simulink model "gm_RLUb_HIL"  (R2018b)
settings: Solver=VariableStepAuto  StartTime=0.0  StopTime=15e-3  RelTol=1e-6  EnableMultiTasking=on
undefined symbols (not defined in the file or in its folder): dt, I_FS, L, R, U_FS
libraries: simulink x53, hdlmdlgenlib x11, hdlsllib x9
settings Model: Creator=suti  LastModifiedBy=natlo
settings DataIOCC: LimitDataPoints=on  SaveFormat=Array  SaveOutput=off  SaveTime=off
settings OptimizationCC: BlockReduction=off  ConditionallyExecuteInputs=off  DefaultParameterBehavior=Inlined  ExpressionDepthLimit=2147483647  LifeSpan=1
settings DebuggingCC: AlgebraicLoopMsg=error  UnderspecifiedInitializationDetection=Classic  MergeDetectMultiDrivingBlocksExec=none  SolverPrmCheckMsg=warning  InheritedTsInSrcMsg=none  FcnCallInpInsideContextMsg=warning  StateNameClashWarn=warning  SFUnexpectedBacktrackingDiag=warning  SFNoUnconditionalDefaultTransitionDiag=warning  SFExecutionAtInitializationDiag=none
settings HardwareCC: ProdBitPerPointer=32  ProdBitPerSizeT=32  ProdBitPerPtrDiffT=32  ProdLargestAtomicFloat=None  ProdIntDivRoundTo=Undefined  ProdEndianess=Unspecified  ProdWordSize=32  ProdHWDeviceType=ASIC/FPGA->ASIC/FPGA  TargetBitPerPointer=64  TargetBitPerSizeT=64  TargetBitPerPtrDiffT=64  TargetLongLongMode=on  TargetIntDivRoundTo=Zero  TargetEndianess=LittleEndian  TargetWordSize=64  TargetHWDeviceType=Custom Processor->MATLAB Host Computer  ProdEqTarget=off
settings ModelReferenceCC: PropagateSignalLabelsOutOfModel=off
settings SFSimCC: SimUseLocalCustomCode=off
settings RTWCC: RTWUseLocalCustomCode=off
settings CodeAppCC: StateflowObjectComments=on
settings GRTTargetCC: TargetLangStandard=C89/C90 (ANSI)  GeneratePreprocessorConditionals=Disable all  CombineOutputUpdateFcns=off  GRTInterface=on
settings ConfigComp: CovMetricSettings=dw  CovHtmlReporting=on  CovSaveCumulativeToWorkspaceVar=on  CovSaveSingleToWorkspaceVar=on  CovExternalEMLEnable=off  CovSFcnEnable=off

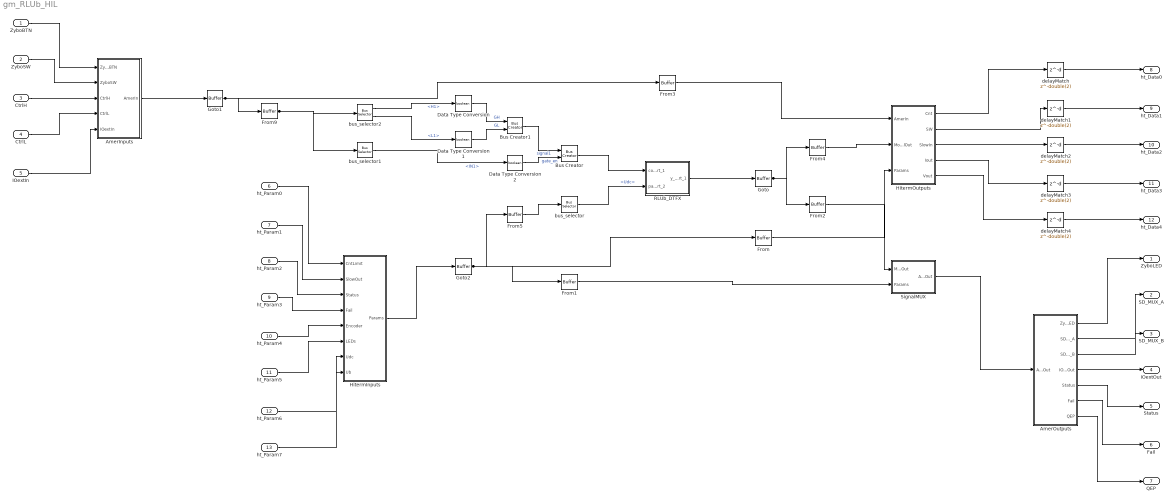
== system gm_RLUb_HIL ==
  ZyboBTN : Inport  OutDataTypeStr=fixdt(0, 3, 0)  PortDimensions=1  SampleTime=5e-08
  ZyboSW : Inport  Port=2  OutDataTypeStr=fixdt(0, 4, 0)  PortDimensions=1  SampleTime=5e-08
  CtrlH : Inport  Port=3  OutDataTypeStr=fixdt(0, 4, 0)  PortDimensions=1  SampleTime=5e-08
  CtrlL : Inport  Port=4  OutDataTypeStr=fixdt(0, 4, 0)  PortDimensions=1  SampleTime=5e-08
  IOextIn : Inport  Port=5  OutDataTypeStr=uint8  PortDimensions=1  SampleTime=5e-08
  ht_Param0 : Inport  Port=6  OutDataTypeStr=uint32  PortDimensions=1  SampleTime=5e-08
  ht_Param1 : Inport  Port=7  OutDataTypeStr=uint32  PortDimensions=1  SampleTime=5e-08
  ht_Param2 : Inport  Port=8  OutDataTypeStr=uint32  PortDimensions=1  SampleTime=5e-08
  ht_Param3 : Inport  Port=9  OutDataTypeStr=uint32  PortDimensions=1  SampleTime=5e-08
  ht_Param4 : Inport  Port=10  OutDataTypeStr=uint32  PortDimensions=1  SampleTime=5e-08
  ht_Param5 : Inport  Port=11  OutDataTypeStr=uint32  PortDimensions=1  SampleTime=5e-08
  ht_Param6 : Inport  Port=12  OutDataTypeStr=uint32  PortDimensions=1  SampleTime=5e-08
  ht_Param7 : Inport  Port=13  OutDataTypeStr=uint32  PortDimensions=1  SampleTime=5e-08
  AmerInputs : Subsystem
  AmerOutputs : Subsystem
  Bus Creator : BusCreator  Inputs=2
  Bus Creator1 : BusCreator  Inputs=2
  Data Type Conversion : DataTypeConversion  OutDataTypeStr=boolean  SampleTime=5e-08
  Data Type Conversion1 : DataTypeConversion  OutDataTypeStr=boolean  SampleTime=5e-08
  Data Type Conversion2 : DataTypeConversion  OutDataTypeStr=boolean  SampleTime=5e-08
  From{,1..5,9} (7 alike) : hdlmdlgenlib/Buffer
      settings: SourceProductName=HDL Coder  SourceProductBaseCode=HD
  Goto : hdlmdlgenlib/Buffer
      settings: SourceProductName=HDL Coder  SourceProductBaseCode=HD
  Goto1 : hdlmdlgenlib/Buffer
      settings: SourceProductName=HDL Coder  SourceProductBaseCode=HD
  Goto2 : hdlmdlgenlib/Buffer
      settings: SourceProductName=HDL Coder  SourceProductBaseCode=HD
  HitermInputs : Subsystem
  HitermOutputs : Subsystem
  RLUb_DTFX : Subsystem
  SignalMUX : Subsystem
  bus_selector : BusSelector  OutputSignals=Udc,Ub  OutputAsBus=on
  bus_selector1 : BusSelector  OutputSignals=SlowIn.IN1  OutputAsBus=on
  bus_selector2 : BusSelector  OutputSignals=Ctrl.GH.H1,Ctrl.GL.L1
  delayMatch{,1..4} (5 alike) : Delay  DelayLength=double(2)  InitialCondition=0  InputProcessing=Inherited  SampleTime=5e-08
  ZyboLED : Outport  SampleTime=dt
  SD_MUX_A : Outport  Port=2  SampleTime=dt
  SD_MUX_B : Outport  Port=3  SampleTime=dt
  IOextOut : Outport  Port=4
  Status : Outport  Port=5
  Fail : Outport  Port=6
  QEP : Outport  Port=7
  ht_Data0 : Outport  Port=8
  ht_Data1 : Outport  Port=9
  ht_Data2 : Outport  Port=10
  ht_Data3 : Outport  Port=11
  ht_Data4 : Outport  Port=12
  wires:
  ZyboBTN/1 -> AmerInputs/1(ZyboBTN)
  ZyboSW/1 -> AmerInputs/2(ZyboSW)
  CtrlH/1 -> AmerInputs/3(CtrlH)
  CtrlL/1 -> AmerInputs/4(CtrlL)
  IOextIn/1 -> AmerInputs/5(IOextIn)
  ht_Param0/1 -> HitermInputs/1(CntLimit)
  ht_Param1/1 -> HitermInputs/2(SlowOut)
  ht_Param2/1 -> HitermInputs/3(Status)
  ht_Param3/1 -> HitermInputs/4(Fail)
  ht_Param4/1 -> HitermInputs/5(Encoder)
  ht_Param5/1 -> HitermInputs/6(LEDs)
  ht_Param6/1 -> HitermInputs/7(Udc)
  ht_Param7/1 -> HitermInputs/8(Ub)
  AmerInputs/1(AmerIn) -> Goto1/1
  AmerOutputs/1(ZyboLED) -> ZyboLED/1
  AmerOutputs/2(SD_MUX_A) -> SD_MUX_A/1
  AmerOutputs/3(SD_MUX_B) -> SD_MUX_B/1
  AmerOutputs/4(IOextOut) -> IOextOut/1
  AmerOutputs/5(Status) -> Status/1
  AmerOutputs/6(Fail) -> Fail/1
  AmerOutputs/7(QEP) -> QEP/1
  Bus Creator/1 -> RLUb_DTFX/1(control_Inport_1)
  Bus Creator1/1 -> Bus Creator/1  "signal1"
  bus_selector/1 -> RLUb_DTFX/2(par_Inport_2)  "<Udc>"
  bus_selector1/1 -> Data Type Conversion2/1  "<IN1>"
  bus_selector2/1 -> Data Type Conversion/1  "<H1>"
  bus_selector2/2 -> Data Type Conversion1/1  "<L1>"
  Data Type Conversion/1 -> Bus Creator1/1  "GH"
  Data Type Conversion1/1 -> Bus Creator1/2  "GL"
  Data Type Conversion2/1 -> Bus Creator/2  "gate_en"
  From/1 -> HitermOutputs/3(Params)
  From1/1 -> SignalMUX/2(Params)
  From2/1 -> SignalMUX/1(ModelOut)
  From3/1 -> HitermOutputs/1(AmerIn)
  From4/1 -> HitermOutputs/2(ModelOut)
  From5/1 -> bus_selector/1
  From9/1 -> bus_selector2/1, bus_selector1/1
  HitermInputs/1(Params) -> Goto2/1
  delayMatch/1 -> ht_Data0/1
  delayMatch1/1 -> ht_Data1/1
  delayMatch2/1 -> ht_Data2/1
  delayMatch3/1 -> ht_Data3/1
  delayMatch4/1 -> ht_Data4/1
  RLUb_DTFX/1(y_Outport_1) -> Goto/1
  SignalMUX/1(AmerOut) -> AmerOutputs/1(AmerOut)
  Goto2/1 -> From5/1, From1/1, From/1
  Goto/1 -> From4/1, From2/1
  Goto1/1 -> From9/1, From3/1
  HitermOutputs/1(Cnt) -> delayMatch/1
  HitermOutputs/2(SW) -> delayMatch1/1
  HitermOutputs/3(SlowIn) -> delayMatch2/1
  HitermOutputs/4(Iout) -> delayMatch3/1
  HitermOutputs/5(Vout) -> delayMatch4/1

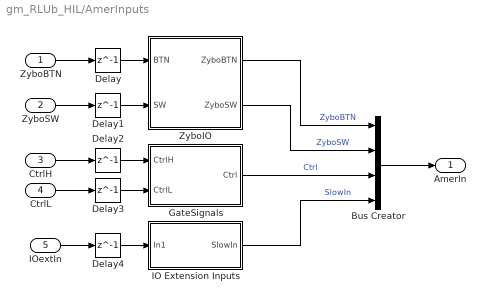
== system gm_RLUb_HIL/AmerInputs ==
  ZyboBTN : Inport  OutDataTypeStr=fixdt(0, 3, 0)  PortDimensions=1  SampleTime=5e-08
  ZyboSW : Inport  Port=2  OutDataTypeStr=fixdt(0, 4, 0)  PortDimensions=1  SampleTime=5e-08
  CtrlH : Inport  Port=3  OutDataTypeStr=fixdt(0, 4, 0)  PortDimensions=1  SampleTime=5e-08
  CtrlL : Inport  Port=4  OutDataTypeStr=fixdt(0, 4, 0)  PortDimensions=1  SampleTime=5e-08
  IOextIn : Inport  Port=5  OutDataTypeStr=uint8  PortDimensions=1  SampleTime=5e-08
  Bus Creator : BusCreator  Inputs=4
  Delay{,1..4} (5 alike) : Delay  DelayLength=1  InitialCondition=0
  GateSignals : Subsystem
  IO Extension Inputs : Subsystem
  ZyboIO : Subsystem
  AmerIn : Outport
  wires:
  Bus Creator/1 -> AmerIn/1
  Delay/1 -> ZyboIO/1(BTN)
  Delay1/1 -> ZyboIO/2(SW)
  Delay2/1 -> GateSignals/1(CtrlH)
  Delay3/1 -> GateSignals/2(CtrlL)
  Delay4/1 -> IO Extension Inputs/1(In1)
  GateSignals/1(Ctrl) -> Bus Creator/3  "Ctrl"
  IO Extension Inputs/1(SlowIn) -> Bus Creator/4  "SlowIn"
  ZyboIO/1(ZyboBTN) -> Bus Creator/1  "ZyboBTN"
  ZyboIO/2(ZyboSW) -> Bus Creator/2  "ZyboSW"
  ZyboBTN/1 -> Delay/1
  ZyboSW/1 -> Delay1/1
  CtrlH/1 -> Delay2/1
  CtrlL/1 -> Delay3/1
  IOextIn/1 -> Delay4/1

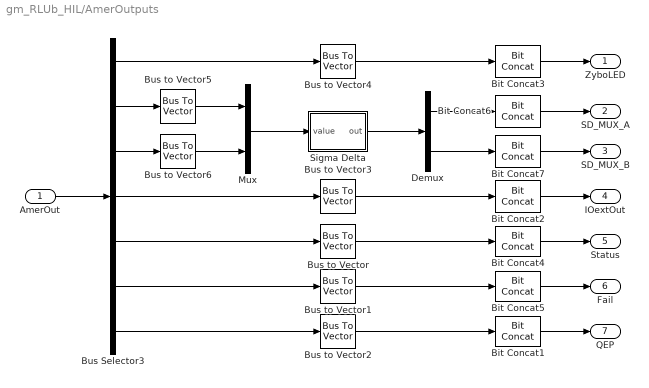
== system gm_RLUb_HIL/AmerOutputs ==
  AmerOut : Inport  SampleTime=5e-08
  Bit Concat{1..7} (7 alike) : hdlsllib/Logic and Bit Operations/Bit Concat  numInputs=1
      settings: SourceProductName=HDL Coder  SourceProductBaseCode=HD
  Bus Selector3 : BusSelector  OutputSignals=ZyboLED,ANA,ANB,SlowOut,Status,Fail,Encoder
  Bus to Vector{,1..6} (7 alike) : BusToVector
  Demux : Demux  Outputs=[8,8]
  Mux : Mux  Inputs=2
  Sigma Delta : Subsystem  mask{N=double(16), dt=double(-1)}
      mask prompts: N "Required resolution (bits)"; dt "Sample time"
  ZyboLED : Outport
  SD_MUX_A : Outport  Port=2  SampleTime=dt
  SD_MUX_B : Outport  Port=3  SampleTime=dt
  IOextOut : Outport  Port=4
  Status : Outport  Port=5
  Fail : Outport  Port=6
  QEP : Outport  Port=7
  wires:
  Bit Concat1/1 -> QEP/1
  Bit Concat2/1 -> IOextOut/1
  Bit Concat3/1 -> ZyboLED/1
  Bit Concat4/1 -> Status/1
  Bit Concat5/1 -> Fail/1
  Bit Concat6/1 -> SD_MUX_A/1
  Bit Concat7/1 -> SD_MUX_B/1
  Bus Selector3/1 -> Bus to Vector4/1
  Bus Selector3/2 -> Bus to Vector5/1
  Bus Selector3/3 -> Bus to Vector6/1
  Bus Selector3/4 -> Bus to Vector3/1
  Bus Selector3/5 -> Bus to Vector/1
  Bus Selector3/6 -> Bus to Vector1/1
  Bus Selector3/7 -> Bus to Vector2/1
  Bus to Vector/1 -> Bit Concat4/1
  Bus to Vector1/1 -> Bit Concat5/1
  Bus to Vector2/1 -> Bit Concat1/1
  Bus to Vector3/1 -> Bit Concat2/1
  Bus to Vector4/1 -> Bit Concat3/1
  Bus to Vector5/1 -> Mux/1
  Bus to Vector6/1 -> Mux/2
  Demux/1 -> Bit Concat6/1
  Demux/2 -> Bit Concat7/1
  Mux/1 -> Sigma Delta/1(value)
  Sigma Delta/1(out) -> Demux/1
  AmerOut/1 -> Bus Selector3/1

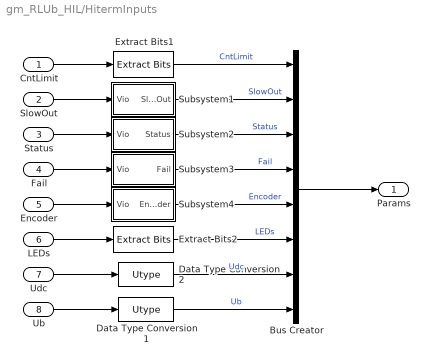
== system gm_RLUb_HIL/HitermInputs ==
  CntLimit : Inport  OutDataTypeStr=uint32  PortDimensions=1  SampleTime=5e-08
  SlowOut : Inport  Port=2  OutDataTypeStr=uint32  PortDimensions=1  SampleTime=5e-08
  Status : Inport  Port=3  OutDataTypeStr=uint32  PortDimensions=1  SampleTime=5e-08
  Fail : Inport  Port=4  OutDataTypeStr=uint32  PortDimensions=1  SampleTime=5e-08
  Encoder : Inport  Port=5  OutDataTypeStr=uint32  PortDimensions=1  SampleTime=5e-08
  LEDs : Inport  Port=6  OutDataTypeStr=uint32  PortDimensions=1  SampleTime=5e-08
  Udc : Inport  Port=7  OutDataTypeStr=uint32  PortDimensions=1  SampleTime=5e-08
  Ub : Inport  Port=8  OutDataTypeStr=uint32  PortDimensions=1  SampleTime=5e-08
  Bus Creator : BusCreator  Inputs=8
  Data Type Conversion1 : DataTypeConversion  OutDataTypeStr=Utype  ConvertRealWorld=Stored Integer (SI)
  Data Type Conversion2 : DataTypeConversion  OutMin=[0]  OutDataTypeStr=Utype  ConvertRealWorld=Stored Integer (SI)
  Extract Bits1 : simulink/Logic and Bit Operations/Extract Bits  bitsToExtract=Range of bits  numBits=8  bitIdxRange=[0 15]  outScalingMode=Treat bit field as an integer
      settings: SourceProductName=Simulink
  Extract Bits2 : simulink/Logic and Bit Operations/Extract Bits  bitsToExtract=Range of bits  numBits=8  bitIdxRange=[0 3]  outScalingMode=Treat bit field as an integer
      settings: SourceProductName=Simulink
  Subsystem1 : Subsystem
  Subsystem2 : Subsystem
  Subsystem3 : Subsystem
  Subsystem4 : Subsystem
  Params : Outport
  wires:
  Bus Creator/1 -> Params/1
  Data Type Conversion1/1 -> Bus Creator/8  "Ub"
  Data Type Conversion2/1 -> Bus Creator/7  "Udc"
  Extract Bits1/1 -> Bus Creator/1  "CntLimit"
  Extract Bits2/1 -> Bus Creator/6  "LEDs"
  Subsystem1/1(SlowOut) -> Bus Creator/2  "SlowOut"
  Subsystem2/1(Status) -> Bus Creator/3  "Status"
  Subsystem3/1(Fail) -> Bus Creator/4  "Fail"
  Subsystem4/1(Encoder) -> Bus Creator/5  "Encoder"
  CntLimit/1 -> Extract Bits1/1
  SlowOut/1 -> Subsystem1/1(Vio)
  Status/1 -> Subsystem2/1(Vio)
  Fail/1 -> Subsystem3/1(Vio)
  Encoder/1 -> Subsystem4/1(Vio)
  LEDs/1 -> Extract Bits2/1
  Udc/1 -> Data Type Conversion2/1
  Ub/1 -> Data Type Conversion1/1

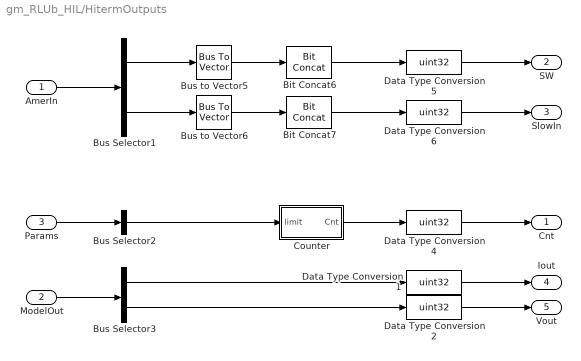
== system gm_RLUb_HIL/HitermOutputs ==
  AmerIn : Inport  SampleTime=5e-08
  ModelOut : Inport  Port=2  SampleTime=5e-08
  Params : Inport  Port=3  SampleTime=5e-08
  Bit Concat6 : hdlsllib/Logic and Bit Operations/Bit Concat  numInputs=1
      settings: SourceProductName=HDL Coder  SourceProductBaseCode=HD
  Bit Concat7 : hdlsllib/Logic and Bit Operations/Bit Concat  numInputs=1
      settings: SourceProductName=HDL Coder  SourceProductBaseCode=HD
  Bus Selector1 : BusSelector  OutputSignals=ZyboSW,SlowIn
  Bus Selector2 : BusSelector  OutputSignals=CntLimit
  Bus Selector3 : BusSelector  OutputSignals=Iout,Vout
  Bus to Vector5 : BusToVector
  Bus to Vector6 : BusToVector
  Counter : Subsystem
  Data Type Conversion1 : DataTypeConversion  OutDataTypeStr=uint32  ConvertRealWorld=Stored Integer (SI)
  Data Type Conversion2 : DataTypeConversion  OutDataTypeStr=uint32  ConvertRealWorld=Stored Integer (SI)
  Data Type Conversion4 : DataTypeConversion  OutDataTypeStr=uint32
  Data Type Conversion5 : DataTypeConversion  OutDataTypeStr=uint32
  Data Type Conversion6 : DataTypeConversion  OutDataTypeStr=uint32
  Cnt : Outport
  SW : Outport  Port=2
  SlowIn : Outport  Port=3
  Iout : Outport  Port=4
  Vout : Outport  Port=5
  wires:
  Bit Concat6/1 -> Data Type Conversion5/1
  Bit Concat7/1 -> Data Type Conversion6/1
  Bus Selector1/1 -> Bus to Vector5/1
  Bus Selector1/2 -> Bus to Vector6/1
  Bus Selector2/1 -> Counter/1(limit)
  Bus Selector3/1 -> Data Type Conversion1/1
  Bus Selector3/2 -> Data Type Conversion2/1
  Bus to Vector5/1 -> Bit Concat6/1
  Bus to Vector6/1 -> Bit Concat7/1
  Counter/1(Cnt) -> Data Type Conversion4/1
  Data Type Conversion1/1 -> Iout/1
  Data Type Conversion2/1 -> Vout/1
  Data Type Conversion4/1 -> Cnt/1
  Data Type Conversion5/1 -> SW/1
  Data Type Conversion6/1 -> SlowIn/1
  AmerIn/1 -> Bus Selector1/1
  ModelOut/1 -> Bus Selector3/1
  Params/1 -> Bus Selector2/1

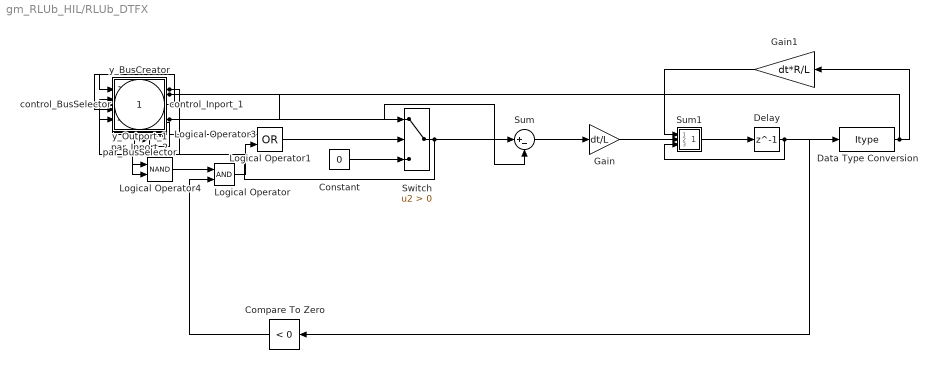
== system gm_RLUb_HIL/RLUb_DTFX ==
  control_Inport_1 : Inport  SampleTime=5e-08
  par_Inport_2 : Inport  Port=2  SampleTime=5e-08
  Compare To Zero : simulink/Logic and Bit Operations/Compare To Zero  relop=<  OutDataTypeStr=boolean
  Constant : Constant  Value=0  OutDataTypeStr=Inherit: Inherit via back propagation  SampleTime=-1
  Data Type Conversion : DataTypeConversion  OutDataTypeStr=Itype
  Delay : Delay  DelayLength=1
  Gain : Gain  Gain=dt/L  OutMax=[2*U_FS*dt/L]  OutDataTypeStr=fixdt(1,vbits)
  Gain1 : Gain  Gain=dt*R/L  OutMax=[I_FS*dt*R/L]  OutDataTypeStr=fixdt(1,vbits)
  Logical Operator : Logic  IconShape=distinctive  AllPortsSameDT=off  OutDataTypeStr=boolean
  Logical Operator1 : Logic  Operator=OR  IconShape=distinctive  AllPortsSameDT=off  OutDataTypeStr=boolean
  Logical Operator3 : Logic  IconShape=distinctive  AllPortsSameDT=off  OutDataTypeStr=boolean
  Logical Operator4 : Logic  Operator=NAND  IconShape=distinctive  AllPortsSameDT=off  OutDataTypeStr=boolean
  Sum : Sum  Inputs=|+-  OutDataTypeStr=Inherit: Same as accumulator
  Sum1 : Subsystem
  Switch : Switch  Criteria=u2 > Threshold
  control_BusSelector : Subsystem
  par_BusSelector : Subsystem
  y_BusCreator : Subsystem
  y_Outport_1 : Outport
  wires:
  Constant/1 -> Switch/3
  Data Type Conversion/1 -> y_BusCreator/1(y_BusCreator_In1), Gain1/1
  Logical Operator3/1 -> Logical Operator1/1
  Logical Operator4/1 -> Logical Operator/1
  Switch/1 -> y_BusCreator/2(y_BusCreator_In2), Sum/1
  control_BusSelector/1(control_BusSelector_Out1) -> Logical Operator4/2, Logical Operator3/2
  control_BusSelector/2(control_BusSelector_Out2) -> Logical Operator3/1
  control_BusSelector/3(control_BusSelector_Out3) -> Logical Operator4/1
  par_BusSelector/1(par_BusSelector_Out1) -> y_BusCreator/3(y_BusCreator_In3), Switch/1
  par_BusSelector/2(par_BusSelector_Out2) -> y_BusCreator/4(y_BusCreator_In4), Sum/2
  y_BusCreator/1(y_BusCreator_Out1) -> y_Outport_1/1
  control_Inport_1/1 -> control_BusSelector/1(control_BusSelector_In1)
  par_Inport_2/1 -> par_BusSelector/1(par_BusSelector_In1)
  Compare To Zero/1 -> Logical Operator/2
  Logical Operator/1 -> Logical Operator1/2
  Logical Operator1/1 -> Switch/2
  Sum/1 -> Gain/1
  Gain/1 -> Sum1/2(In2)
  Gain1/1 -> Sum1/1(In1)
  Sum1/1(Out1) -> Delay/1
  Delay/1 -> Sum1/3(In3), Data Type Conversion/1, Compare To Zero/1

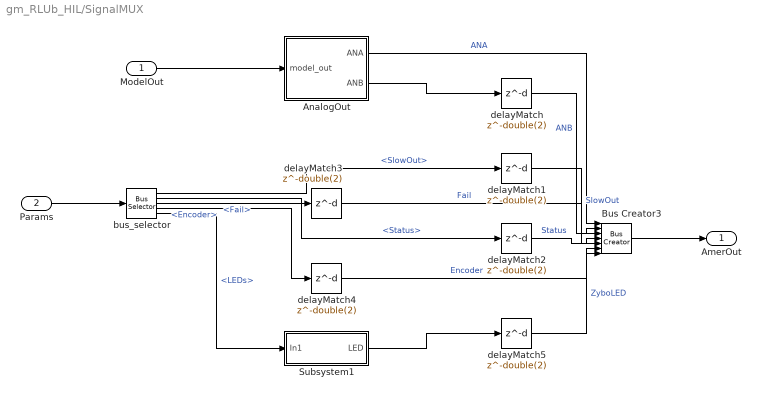
== system gm_RLUb_HIL/SignalMUX ==
  ModelOut : Inport  SampleTime=5e-08
  Params : Inport  Port=2  SampleTime=5e-08
  AnalogOut : Subsystem
  Bus Creator3 : BusCreator  Inputs=7
  Subsystem1 : Subsystem
  bus_selector : BusSelector  OutputSignals=SlowOut,Status,Fail,Encoder,LEDs
  delayMatch{,1..5} (6 alike) : Delay  DelayLength=double(2)  InitialCondition=0  InputProcessing=Inherited  SampleTime=5e-08
  AmerOut : Outport
  wires:
  AnalogOut/1(ANA) -> Bus Creator3/1  "ANA"
  delayMatch/1 -> Bus Creator3/2  "ANB"
  Bus Creator3/1 -> AmerOut/1
  delayMatch1/1 -> Bus Creator3/3  "SlowOut"
  delayMatch2/1 -> Bus Creator3/4  "Status"
  delayMatch3/1 -> Bus Creator3/5  "Fail"
  delayMatch4/1 -> Bus Creator3/6  "Encoder"
  bus_selector/5 -> Subsystem1/1(In1)  "<LEDs>"
  delayMatch5/1 -> Bus Creator3/7  "ZyboLED"
  ModelOut/1 -> AnalogOut/1(model_out)
  Params/1 -> bus_selector/1
  AnalogOut/2(ANB) -> delayMatch/1
  bus_selector/1 -> delayMatch1/1  "<SlowOut>"
  bus_selector/2 -> delayMatch2/1  "<Status>"
  bus_selector/3 -> delayMatch3/1  "<Fail>"
  bus_selector/4 -> delayMatch4/1  "<Encoder>"
  Subsystem1/1(LED) -> delayMatch5/1

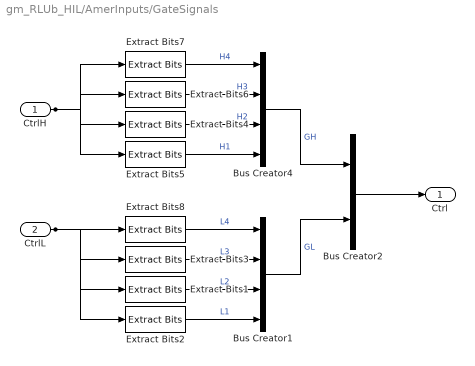
== system gm_RLUb_HIL/AmerInputs/GateSignals ==
  CtrlH : Inport  OutDataTypeStr=fixdt(0, 4, 0)  PortDimensions=1  SampleTime=5e-08
  CtrlL : Inport  Port=2  OutDataTypeStr=fixdt(0, 4, 0)  PortDimensions=1  SampleTime=5e-08
  Bus Creator1 : BusCreator  Inputs=4
  Bus Creator2 : BusCreator  Inputs=2
  Bus Creator4 : BusCreator  Inputs=4
  Extract Bits1 : simulink/Logic and Bit Operations/Extract Bits  bitsToExtract=Range of bits  numBits=8  bitIdxRange=[1 1]  outScalingMode=Treat bit field as an integer
      settings: SourceProductName=Simulink
  Extract Bits2 : simulink/Logic and Bit Operations/Extract Bits  bitsToExtract=Range of bits  numBits=8  bitIdxRange=[0 0]  outScalingMode=Treat bit field as an integer
      settings: SourceProductName=Simulink
  Extract Bits3 : simulink/Logic and Bit Operations/Extract Bits  bitsToExtract=Range of bits  numBits=8  bitIdxRange=[2 2]  outScalingMode=Treat bit field as an integer
      settings: SourceProductName=Simulink
  Extract Bits4 : simulink/Logic and Bit Operations/Extract Bits  bitsToExtract=Range of bits  numBits=8  bitIdxRange=[1 1]  outScalingMode=Treat bit field as an integer
      settings: SourceProductName=Simulink
  Extract Bits5 : simulink/Logic and Bit Operations/Extract Bits  bitsToExtract=Range of bits  numBits=8  bitIdxRange=[0 0]  outScalingMode=Treat bit field as an integer
      settings: SourceProductName=Simulink
  Extract Bits6 : simulink/Logic and Bit Operations/Extract Bits  bitsToExtract=Range of bits  numBits=8  bitIdxRange=[2 2]  outScalingMode=Treat bit field as an integer
      settings: SourceProductName=Simulink
  Extract Bits7 : simulink/Logic and Bit Operations/Extract Bits  bitsToExtract=Range of bits  numBits=8  bitIdxRange=[3 3]  outScalingMode=Treat bit field as an integer
      settings: SourceProductName=Simulink
  Extract Bits8 : simulink/Logic and Bit Operations/Extract Bits  bitsToExtract=Range of bits  numBits=8  bitIdxRange=[3 3]  outScalingMode=Treat bit field as an integer
      settings: SourceProductName=Simulink
  Ctrl : Outport
  wires:
  Bus Creator1/1 -> Bus Creator2/2  "GL"
  Bus Creator2/1 -> Ctrl/1
  Bus Creator4/1 -> Bus Creator2/1  "GH"
  Extract Bits1/1 -> Bus Creator1/3  "L2"
  Extract Bits2/1 -> Bus Creator1/4  "L1"
  Extract Bits3/1 -> Bus Creator1/2  "L3"
  Extract Bits4/1 -> Bus Creator4/3  "H2"
  Extract Bits5/1 -> Bus Creator4/4  "H1"
  Extract Bits6/1 -> Bus Creator4/2  "H3"
  Extract Bits7/1 -> Bus Creator4/1  "H4"
  Extract Bits8/1 -> Bus Creator1/1  "L4"
  CtrlH/1 -> Extract Bits7/1, Extract Bits6/1, Extract Bits5/1, Extract Bits4/1
  CtrlL/1 -> Extract Bits8/1, Extract Bits3/1, Extract Bits2/1, Extract Bits1/1

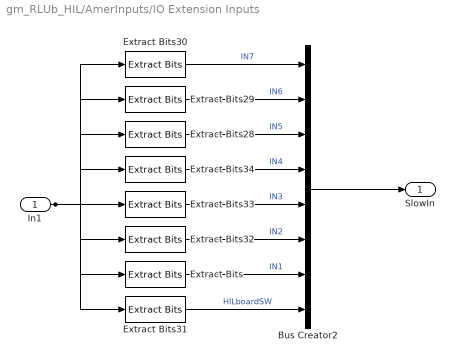
== system gm_RLUb_HIL/AmerInputs/IO Extension Inputs ==
  In1 : Inport  OutDataTypeStr=uint8  PortDimensions=1  SampleTime=5e-08
  Bus Creator2 : BusCreator  Inputs=8
  Extract Bits : simulink/Logic and Bit Operations/Extract Bits  bitsToExtract=Range of bits  numBits=8  bitIdxRange=[1 1]  outScalingMode=Treat bit field as an integer
      settings: SourceProductName=Simulink
  Extract Bits28 : simulink/Logic and Bit Operations/Extract Bits  bitsToExtract=Range of bits  numBits=8  bitIdxRange=[5 5]  outScalingMode=Treat bit field as an integer
      settings: SourceProductName=Simulink
  Extract Bits29 : simulink/Logic and Bit Operations/Extract Bits  bitsToExtract=Range of bits  numBits=8  bitIdxRange=[6 6]  outScalingMode=Treat bit field as an integer
      settings: SourceProductName=Simulink
  Extract Bits30 : simulink/Logic and Bit Operations/Extract Bits  bitsToExtract=Range of bits  numBits=8  bitIdxRange=[7 7]  outScalingMode=Treat bit field as an integer
      settings: SourceProductName=Simulink
  Extract Bits31 : simulink/Logic and Bit Operations/Extract Bits  bitsToExtract=Range of bits  numBits=8  bitIdxRange=[0 0]  outScalingMode=Treat bit field as an integer
      settings: SourceProductName=Simulink
  Extract Bits32 : simulink/Logic and Bit Operations/Extract Bits  bitsToExtract=Range of bits  numBits=8  bitIdxRange=[2 2]  outScalingMode=Treat bit field as an integer
      settings: SourceProductName=Simulink
  Extract Bits33 : simulink/Logic and Bit Operations/Extract Bits  bitsToExtract=Range of bits  numBits=8  bitIdxRange=[3 3]  outScalingMode=Treat bit field as an integer
      settings: SourceProductName=Simulink
  Extract Bits34 : simulink/Logic and Bit Operations/Extract Bits  bitsToExtract=Range of bits  numBits=8  bitIdxRange=[4 4]  outScalingMode=Treat bit field as an integer
      settings: SourceProductName=Simulink
  SlowIn : Outport
  wires:
  Bus Creator2/1 -> SlowIn/1
  Extract Bits/1 -> Bus Creator2/7  "IN1"
  Extract Bits28/1 -> Bus Creator2/3  "IN5"
  Extract Bits29/1 -> Bus Creator2/2  "IN6"
  Extract Bits30/1 -> Bus Creator2/1  "IN7"
  Extract Bits31/1 -> Bus Creator2/8  "HILboardSW"
  Extract Bits32/1 -> Bus Creator2/6  "IN2"
  Extract Bits33/1 -> Bus Creator2/5  "IN3"
  Extract Bits34/1 -> Bus Creator2/4  "IN4"
  In1/1 -> Extract Bits34/1, Extract Bits33/1, Extract Bits32/1, Extract Bits31/1, Extract Bits30/1, Extract Bits29/1, Extract Bits28/1, Extract Bits/1

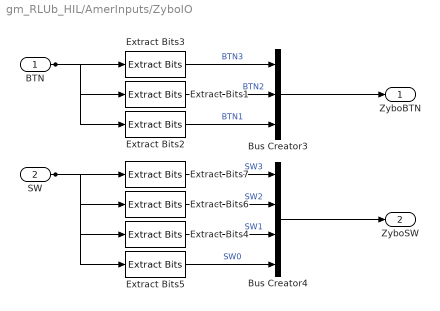
== system gm_RLUb_HIL/AmerInputs/ZyboIO ==
  BTN : Inport  OutDataTypeStr=fixdt(0, 3, 0)  PortDimensions=1  SampleTime=5e-08
  SW : Inport  Port=2  OutDataTypeStr=fixdt(0, 4, 0)  PortDimensions=1  SampleTime=5e-08
  Bus Creator3 : BusCreator  Inputs=3
  Bus Creator4 : BusCreator  Inputs=4
  Extract Bits1 : simulink/Logic and Bit Operations/Extract Bits  bitsToExtract=Range of bits  numBits=8  bitIdxRange=[1 1]  outScalingMode=Treat bit field as an integer
      settings: SourceProductName=Simulink
  Extract Bits2 : simulink/Logic and Bit Operations/Extract Bits  bitsToExtract=Range of bits  numBits=8  bitIdxRange=[0 0]  outScalingMode=Treat bit field as an integer
      settings: SourceProductName=Simulink
  Extract Bits3 : simulink/Logic and Bit Operations/Extract Bits  bitsToExtract=Range of bits  numBits=8  bitIdxRange=[2 2]  outScalingMode=Treat bit field as an integer
      settings: SourceProductName=Simulink
  Extract Bits4 : simulink/Logic and Bit Operations/Extract Bits  bitsToExtract=Range of bits  numBits=8  bitIdxRange=[1 1]  outScalingMode=Treat bit field as an integer
      settings: SourceProductName=Simulink
  Extract Bits5 : simulink/Logic and Bit Operations/Extract Bits  bitsToExtract=Range of bits  numBits=8  bitIdxRange=[0 0]  outScalingMode=Treat bit field as an integer
      settings: SourceProductName=Simulink
  Extract Bits6 : simulink/Logic and Bit Operations/Extract Bits  bitsToExtract=Range of bits  numBits=8  bitIdxRange=[2 2]  outScalingMode=Treat bit field as an integer
      settings: SourceProductName=Simulink
  Extract Bits7 : simulink/Logic and Bit Operations/Extract Bits  bitsToExtract=Range of bits  numBits=8  bitIdxRange=[3 3]  outScalingMode=Treat bit field as an integer
      settings: SourceProductName=Simulink
  ZyboBTN : Outport
  ZyboSW : Outport  Port=2
  wires:
  Bus Creator3/1 -> ZyboBTN/1
  Bus Creator4/1 -> ZyboSW/1
  Extract Bits1/1 -> Bus Creator3/2  "BTN2"
  Extract Bits2/1 -> Bus Creator3/3  "BTN1"
  Extract Bits3/1 -> Bus Creator3/1  "BTN3"
  Extract Bits4/1 -> Bus Creator4/3  "SW1"
  Extract Bits5/1 -> Bus Creator4/4  "SW0"
  Extract Bits6/1 -> Bus Creator4/2  "SW2"
  Extract Bits7/1 -> Bus Creator4/1  "SW3"
  BTN/1 -> Extract Bits3/1, Extract Bits2/1, Extract Bits1/1
  SW/1 -> Extract Bits7/1, Extract Bits6/1, Extract Bits5/1, Extract Bits4/1

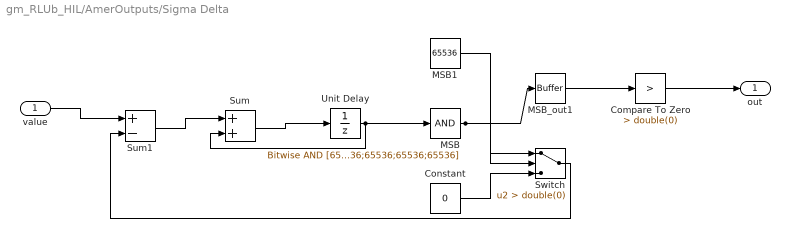
== system gm_RLUb_HIL/AmerOutputs/Sigma Delta ==
  value : Inport  OutDataTypeStr=uint16  PortDimensions=[16]  SampleTime=5e-08
  Compare To Zero : simulink/Logic and Bit Operations/Compare To Constant  relop=>  const=double(0)  OutDataTypeStr=boolean
  Constant : Constant  Value=0  OutDataTypeStr=fixdt(0, 17, 0)  SampleTime=-1
  MSB : simulink/Logic and Bit Operations/Bitwise Operator  logicop=AND  UseBitMask=on  BitMask=[65536;65536;65536;65536;65536;65536;65536;65536;65536;65536;65536;65536;65536;65536;65536;65536]  BitMaskRealWorld=Real World Value
  MSB1 : Constant  Value=65536  OutDataTypeStr=fixdt(0, 17, 0)  SampleTime=-1
  MSB_out1 : hdlmdlgenlib/Buffer
      settings: SourceProductName=HDL Coder  SourceProductBaseCode=HD
  Sum : Sum  AccumDataTypeStr=fixdt(0, 17, 0)  OutDataTypeStr=fixdt(0, 17, 0)  SampleTime=5e-08
  Sum1 : Sum  Inputs=+-  AccumDataTypeStr=fixdt(0, 17, 0)  OutDataTypeStr=fixdt(0, 17, 0)  SampleTime=5e-08
  Switch : Switch  Criteria=u2 > Threshold  Threshold=double(0)  OutDataTypeStr=fixdt(0, 17, 0)  SampleTime=5e-08
  Unit Delay : UnitDelay  InitialCondition=fi(0,0,17,0,'hex','00000')  SampleTime=5e-08
  out : Outport  OutDataTypeStr=boolean
  wires:
  Compare To Zero/1 -> out/1
  Constant/1 -> Switch/3
  MSB_out1/1 -> Compare To Zero/1
  MSB1/1 -> Switch/1
  value/1 -> Sum1/1
  Switch/1 -> Sum1/2
  Sum1/1 -> Sum/1
  Sum/1 -> Unit Delay/1
  Unit Delay/1 -> Sum/2, MSB/1
  MSB/1 -> MSB_out1/1, Switch/2

== system gm_RLUb_HIL/HitermInputs/Subsystem1 ==
  Vio : Inport  OutDataTypeStr=uint32  PortDimensions=1  SampleTime=5e-08
  Bus Creator3 : BusCreator  Inputs=8
  Extract Bits1 : simulink/Logic and Bit Operations/Extract Bits  bitsToExtract=Range of bits  numBits=8  bitIdxRange=[4 4]  outScalingMode=Treat bit field as an integer
      settings: SourceProductName=Simulink
  Extract Bits10 : simulink/Logic and Bit Operations/Extract Bits  bitsToExtract=Range of bits  numBits=8  bitIdxRange=[1 1]  outScalingMode=Treat bit field as an integer
      settings: SourceProductName=Simulink
  Extract Bits2 : simulink/Logic and Bit Operations/Extract Bits  bitsToExtract=Range of bits  numBits=8  bitIdxRange=[5 5]  outScalingMode=Treat bit field as an integer
      settings: SourceProductName=Simulink
  Extract Bits21 : simulink/Logic and Bit Operations/Extract Bits  bitsToExtract=Range of bits  numBits=8  bitIdxRange=[0 0]  outScalingMode=Treat bit field as an integer
      settings: SourceProductName=Simulink
  Extract Bits3 : simulink/Logic and Bit Operations/Extract Bits  bitsToExtract=Range of bits  numBits=8  bitIdxRange=[6 6]  outScalingMode=Treat bit field as an integer
      settings: SourceProductName=Simulink
  Extract Bits4 : simulink/Logic and Bit Operations/Extract Bits  bitsToExtract=Range of bits  numBits=8  bitIdxRange=[7 7]  outScalingMode=Treat bit field as an integer
      settings: SourceProductName=Simulink
  Extract Bits8 : simulink/Logic and Bit Operations/Extract Bits  bitsToExtract=Range of bits  numBits=8  bitIdxRange=[3 3]  outScalingMode=Treat bit field as an integer
      settings: SourceProductName=Simulink
  Extract Bits9 : simulink/Logic and Bit Operations/Extract Bits  bitsToExtract=Range of bits  numBits=8  bitIdxRange=[2 2]  outScalingMode=Treat bit field as an integer
      settings: SourceProductName=Simulink
  SlowOut : Outport
  wires:
  Bus Creator3/1 -> SlowOut/1
  Extract Bits1/1 -> Bus Creator3/4  "OUT4"
  Extract Bits10/1 -> Bus Creator3/7  "OUT1"
  Extract Bits2/1 -> Bus Creator3/3  "OUT5"
  Extract Bits21/1 -> Bus Creator3/8  "HILboardRLED"
  Extract Bits3/1 -> Bus Creator3/2  "OUT6"
  Extract Bits4/1 -> Bus Creator3/1  "OUT7"
  Extract Bits8/1 -> Bus Creator3/5  "OUT3"
  Extract Bits9/1 -> Bus Creator3/6  "OUT2"
  Vio/1 -> Extract Bits9/1, Extract Bits8/1, Extract Bits4/1, Extract Bits3/1, Extract Bits21/1, Extract Bits2/1, Extract Bits10/1, Extract Bits1/1

== system gm_RLUb_HIL/HitermInputs/Subsystem2 ==
  Vio : Inport  OutDataTypeStr=uint32  PortDimensions=1  SampleTime=5e-08
  Bus Creator3 : BusCreator  Inputs=4
  Extract Bits10 : simulink/Logic and Bit Operations/Extract Bits  bitsToExtract=Range of bits  numBits=8  bitIdxRange=[1 1]  outScalingMode=Treat bit field as an integer
      settings: SourceProductName=Simulink
  Extract Bits21 : simulink/Logic and Bit Operations/Extract Bits  bitsToExtract=Range of bits  numBits=8  bitIdxRange=[0 0]  outScalingMode=Treat bit field as an integer
      settings: SourceProductName=Simulink
  Extract Bits8 : simulink/Logic and Bit Operations/Extract Bits  bitsToExtract=Range of bits  numBits=8  bitIdxRange=[3 3]  outScalingMode=Treat bit field as an integer
      settings: SourceProductName=Simulink
  Extract Bits9 : simulink/Logic and Bit Operations/Extract Bits  bitsToExtract=Range of bits  numBits=8  bitIdxRange=[2 2]  outScalingMode=Treat bit field as an integer
      settings: SourceProductName=Simulink
  Status : Outport
  wires:
  Bus Creator3/1 -> Status/1
  Extract Bits10/1 -> Bus Creator3/3  "Status2"
  Extract Bits21/1 -> Bus Creator3/4  "Status1"
  Extract Bits8/1 -> Bus Creator3/1  "Status4"
  Extract Bits9/1 -> Bus Creator3/2  "Status3"
  Vio/1 -> Extract Bits9/1, Extract Bits8/1, Extract Bits21/1, Extract Bits10/1

== system gm_RLUb_HIL/HitermInputs/Subsystem3 ==
  Vio : Inport  OutDataTypeStr=uint32  PortDimensions=1  SampleTime=5e-08
  Bus Creator3 : BusCreator  Inputs=4
  Extract Bits10 : simulink/Logic and Bit Operations/Extract Bits  bitsToExtract=Range of bits  numBits=8  bitIdxRange=[1 1]  outScalingMode=Treat bit field as an integer
      settings: SourceProductName=Simulink
  Extract Bits21 : simulink/Logic and Bit Operations/Extract Bits  bitsToExtract=Range of bits  numBits=8  bitIdxRange=[0 0]  outScalingMode=Treat bit field as an integer
      settings: SourceProductName=Simulink
  Extract Bits8 : simulink/Logic and Bit Operations/Extract Bits  bitsToExtract=Range of bits  numBits=8  bitIdxRange=[3 3]  outScalingMode=Treat bit field as an integer
      settings: SourceProductName=Simulink
  Extract Bits9 : simulink/Logic and Bit Operations/Extract Bits  bitsToExtract=Range of bits  numBits=8  bitIdxRange=[2 2]  outScalingMode=Treat bit field as an integer
      settings: SourceProductName=Simulink
  Fail : Outport
  wires:
  Bus Creator3/1 -> Fail/1
  Extract Bits10/1 -> Bus Creator3/3  "Fail2"
  Extract Bits21/1 -> Bus Creator3/4  "Fail1"
  Extract Bits8/1 -> Bus Creator3/1  "Fail4"
  Extract Bits9/1 -> Bus Creator3/2  "Fail3"
  Vio/1 -> Extract Bits9/1, Extract Bits8/1, Extract Bits21/1, Extract Bits10/1

== system gm_RLUb_HIL/HitermInputs/Subsystem4 ==
  Vio : Inport  OutDataTypeStr=uint32  PortDimensions=1  SampleTime=5e-08
  Bus Creator3 : BusCreator  Inputs=4
  Extract Bits10 : simulink/Logic and Bit Operations/Extract Bits  bitsToExtract=Range of bits  numBits=8  bitIdxRange=[1 1]  outScalingMode=Treat bit field as an integer
      settings: SourceProductName=Simulink
  Extract Bits21 : simulink/Logic and Bit Operations/Extract Bits  bitsToExtract=Range of bits  numBits=8  bitIdxRange=[0 0]  outScalingMode=Treat bit field as an integer
      settings: SourceProductName=Simulink
  Extract Bits8 : simulink/Logic and Bit Operations/Extract Bits  bitsToExtract=Range of bits  numBits=8  bitIdxRange=[3 3]  outScalingMode=Treat bit field as an integer
      settings: SourceProductName=Simulink
  Extract Bits9 : simulink/Logic and Bit Operations/Extract Bits  bitsToExtract=Range of bits  numBits=8  bitIdxRange=[2 2]  outScalingMode=Treat bit field as an integer
      settings: SourceProductName=Simulink
  Encoder : Outport
  wires:
  Bus Creator3/1 -> Encoder/1
  Extract Bits10/1 -> Bus Creator3/3  "B"
  Extract Bits21/1 -> Bus Creator3/4  "A"
  Extract Bits8/1 -> Bus Creator3/1  "I"
  Extract Bits9/1 -> Bus Creator3/2  "Z"
  Vio/1 -> Extract Bits9/1, Extract Bits8/1, Extract Bits21/1, Extract Bits10/1

== system gm_RLUb_HIL/HitermOutputs/Counter ==
  limit : Inport  OutDataTypeStr=uint16  PortDimensions=1  SampleTime=5e-08
  Constant2 : Constant  Value=0  OutDataTypeStr=Inherit: Inherit via back propagation  SampleTime=-1
  Increment Stored Integer : simulink/Additional Math & Discrete/Additional Math: Increment - Decrement/Increment Stored Integer
      settings: SourceProductName=Simulink
  Relational Operator : RelationalOperator  Operator=<=  OutDataTypeStr=boolean  RndMeth=Nearest
  Switch : Switch  Criteria=u2 > Threshold
  Unit Delay : UnitDelay  SampleTime=-1
  Cnt : Outport
  wires:
  Constant2/1 -> Switch/1
  Unit Delay/1 -> Cnt/1, Increment Stored Integer/1
  limit/1 -> Relational Operator/1
  Increment Stored Integer/1 -> Switch/3, Relational Operator/2
  Relational Operator/1 -> Switch/2
  Switch/1 -> Unit Delay/1

== system gm_RLUb_HIL/RLUb_DTFX/Sum1 ==
  In1 : Inport  OutDataTypeStr=fixdt('sfix25_En34')
  In2 : Inport  Port=2  OutDataTypeStr=fixdt('sfix25_En29')
  In3 : Inport  Port=3  OutDataTypeStr=fixdt('sfix42_En34')
  Sum2 : Sum  Inputs=-+  AccumDataTypeStr=fixdt(1,43,34)  OutDataTypeStr=fixdt(1,43,34)
  Sum3 : Sum  AccumDataTypeStr=fixdt(1,43,34)  OutDataTypeStr=fixdt(1,42,34)
  Out1 : Outport
  wires:
  In1/1 -> Sum2/1
  In2/1 -> Sum2/2
  Sum2/1 -> Sum3/1
  In3/1 -> Sum3/2
  Sum3/1 -> Out1/1

== system gm_RLUb_HIL/RLUb_DTFX/control_BusSelector ==
  control_BusSelector_In1 : Inport  SampleTime=5e-08
  control_BusSelector_BusSelector1 : BusSelector  DisableCoverage=on  OutputSignals=gate_en,signal1.GH,signal1.GL
  control_BusSelector_Out1 : Outport
  control_BusSelector_Out2 : Outport  Port=2
  control_BusSelector_Out3 : Outport  Port=3
  wires:
  control_BusSelector_BusSelector1/1 -> control_BusSelector_Out1/1
  control_BusSelector_BusSelector1/2 -> control_BusSelector_Out2/1
  control_BusSelector_BusSelector1/3 -> control_BusSelector_Out3/1
  control_BusSelector_In1/1 -> control_BusSelector_BusSelector1/1

== system gm_RLUb_HIL/RLUb_DTFX/par_BusSelector ==
  par_BusSelector_In1 : Inport  SampleTime=5e-08
  par_BusSelector_BusSelector1 : BusSelector  DisableCoverage=on  OutputSignals=Udc,Ub
  par_BusSelector_Out1 : Outport
  par_BusSelector_Out2 : Outport  Port=2
  wires:
  par_BusSelector_BusSelector1/1 -> par_BusSelector_Out1/1
  par_BusSelector_BusSelector1/2 -> par_BusSelector_Out2/1
  par_BusSelector_In1/1 -> par_BusSelector_BusSelector1/1

== system gm_RLUb_HIL/RLUb_DTFX/y_BusCreator ==
  y_BusCreator_In1 : Inport  OutDataTypeStr=fixdt(1, 25, 17)  PortDimensions=1  SampleTime=5e-08
  y_BusCreator_In2 : Inport  Port=2  OutDataTypeStr=fixdt(1, 25, 16)  PortDimensions=1  SampleTime=5e-08
  y_BusCreator_In3 : Inport  Port=3  OutDataTypeStr=fixdt(1, 25, 16)  PortDimensions=1  SampleTime=5e-08
  y_BusCreator_In4 : Inport  Port=4  OutDataTypeStr=fixdt(1, 25, 16)  PortDimensions=1  SampleTime=5e-08
  y_BusCreator_BusCreator1 : BusCreator  DisableCoverage=on  Inputs='Iout','Vout','Udc','Ub'
  y_BusCreator_Out1 : Outport
  wires:
  y_BusCreator_BusCreator1/1 -> y_BusCreator_Out1/1
  y_BusCreator_In1/1 -> y_BusCreator_BusCreator1/1  "Iout"
  y_BusCreator_In2/1 -> y_BusCreator_BusCreator1/2  "Vout"
  y_BusCreator_In3/1 -> y_BusCreator_BusCreator1/3  "Udc"
  y_BusCreator_In4/1 -> y_BusCreator_BusCreator1/4  "Ub"

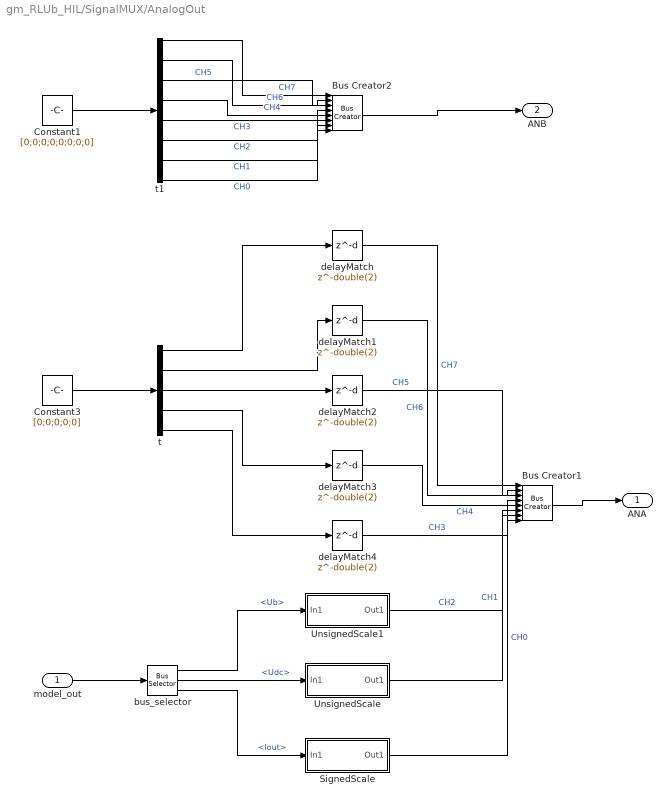
== system gm_RLUb_HIL/SignalMUX/AnalogOut ==
  model_out : Inport  SampleTime=5e-08
  Bus Creator1 : BusCreator  Inputs=8
  Bus Creator2 : BusCreator  Inputs=8
  Constant1 : Constant  Value=[0;0;0;0;0;0;0;0]  OutDataTypeStr=uint16  SampleTime=-1
  Constant3 : Constant  Value=[0;0;0;0;0]  OutDataTypeStr=uint16  SampleTime=-1
  SignedScale : Subsystem  mask{N=double(16), FS=double(62.5)}
      mask prompts: N "Data width"; FS "Full scale"
  UnsignedScale : Subsystem  mask{N=double(16), FS=double(125)}
      mask prompts: N "Data width"; FS "Full scale"
  UnsignedScale1 : Subsystem  mask{N=double(16), FS=double(125)}
      mask prompts: N "Data width"; FS "Full scale"
  bus_selector : BusSelector  OutputSignals=Ub,Udc,Iout
  delayMatch{,1..4} (5 alike) : Delay  DelayLength=double(2)  InitialCondition=0  InputProcessing=Inherited  SampleTime=5e-08
  t : Demux  Outputs=5
  t1 : Demux  Outputs=8
  ANA : Outport
  ANB : Outport  Port=2
  wires:
  Bus Creator1/1 -> ANA/1
  Bus Creator2/1 -> ANB/1
  bus_selector/1 -> UnsignedScale1/1(In1)  "<Ub>"
  bus_selector/2 -> UnsignedScale/1(In1)  "<Udc>"
  bus_selector/3 -> SignedScale/1(In1)  "<Iout>"
  Constant1/1 -> t1/1
  Constant3/1 -> t/1
  delayMatch/1 -> Bus Creator1/1  "CH7"
  delayMatch1/1 -> Bus Creator1/2  "CH6"
  delayMatch2/1 -> Bus Creator1/3  "CH5"
  delayMatch3/1 -> Bus Creator1/4  "CH4"
  delayMatch4/1 -> Bus Creator1/5  "CH3"
  SignedScale/1(Out1) -> Bus Creator1/8  "CH0"
  UnsignedScale/1(Out1) -> Bus Creator1/7  "CH1"
  UnsignedScale1/1(Out1) -> Bus Creator1/6  "CH2"
  t/1 -> delayMatch/1
  t/2 -> delayMatch1/1
  t/3 -> delayMatch2/1
  t/4 -> delayMatch3/1
  t/5 -> delayMatch4/1
  t1/1 -> Bus Creator2/1  "CH7"
  t1/2 -> Bus Creator2/2  "CH6"
  t1/3 -> Bus Creator2/3  "CH5"
  t1/4 -> Bus Creator2/4  "CH4"
  t1/5 -> Bus Creator2/5  "CH3"
  t1/6 -> Bus Creator2/6  "CH2"
  t1/7 -> Bus Creator2/7  "CH1"
  t1/8 -> Bus Creator2/8  "CH0"
  model_out/1 -> bus_selector/1

== system gm_RLUb_HIL/SignalMUX/Subsystem1 ==
  In1 : Inport  OutDataTypeStr=fixdt(0, 4, 0)  PortDimensions=1  SampleTime=5e-08
  Bus Creator1 : BusCreator  Inputs=4
  Extract Bits10 : simulink/Logic and Bit Operations/Extract Bits  bitsToExtract=Range of bits  numBits=8  bitIdxRange=[2 2]  outScalingMode=Treat bit field as an integer
      settings: SourceProductName=Simulink
  Extract Bits11 : simulink/Logic and Bit Operations/Extract Bits  bitsToExtract=Range of bits  numBits=8  bitIdxRange=[3 3]  outScalingMode=Treat bit field as an integer
      settings: SourceProductName=Simulink
  Extract Bits8 : simulink/Logic and Bit Operations/Extract Bits  bitsToExtract=Range of bits  numBits=8  bitIdxRange=[1 1]  outScalingMode=Treat bit field as an integer
      settings: SourceProductName=Simulink
  Extract Bits9 : simulink/Logic and Bit Operations/Extract Bits  bitsToExtract=Range of bits  numBits=8  bitIdxRange=[0 0]  outScalingMode=Treat bit field as an integer
      settings: SourceProductName=Simulink
  LED : Outport
  wires:
  Bus Creator1/1 -> LED/1
  Extract Bits10/1 -> Bus Creator1/2  "LED2"
  Extract Bits11/1 -> Bus Creator1/1  "LED3"
  Extract Bits8/1 -> Bus Creator1/3  "LED1"
  Extract Bits9/1 -> Bus Creator1/4  "LED0"
  In1/1 -> Extract Bits9/1, Extract Bits8/1, Extract Bits11/1, Extract Bits10/1

== system gm_RLUb_HIL/SignalMUX/AnalogOut/SignedScale ==
  In1 : Inport  OutDataTypeStr=fixdt(1, 25, 17)  PortDimensions=1  SampleTime=5e-08
  Bias : Sum  AccumDataTypeStr=uint16  OutDataTypeStr=uint16  RndMeth=Nearest  SampleTime=5e-08
  Bias_const_val : Constant  Value=32768  VectorParams1D=off  OutDataTypeStr=uint16  SampleTime=-1
  Data Type Conversion : DataTypeConversion  OutDataTypeStr=uint16  ConvertRealWorld=Stored Integer (SI)  SampleTime=5e-08
  FS : Product  Inputs=**  OutDataTypeStr=fixdt(1, 50, 31)  SampleTime=5e-08
  FS_const : Constant  Value=524.28802490234375  OutDataTypeStr=fixdt(1, 25, 14)  SampleTime=-1
  FS_out_dtc : DataTypeConversion  OutDataTypeStr=int16  SampleTime=5e-08  SaturateOnIntegerOverflow=on
  HwModeRegister : Delay  DelayLength=double(1)  InitialCondition=0  InputProcessing=Inherited  SampleTime=5e-08
  HwModeRegister1 : Delay  DelayLength=double(1)  InitialCondition=0  InputProcessing=Inherited  SampleTime=5e-08
  PipelineRegister : Delay  DelayLength=double(1)  InitialCondition=0  InputProcessing=Inherited  SampleTime=5e-08
  Out1 : Outport
  wires:
  Bias/1 -> Out1/1
  Data Type Conversion/1 -> Bias/1
  FS_out_dtc/1 -> Data Type Conversion/1
  Bias_const_val/1 -> Bias/2
  FS_const/1 -> HwModeRegister/1
  PipelineRegister/1 -> FS_out_dtc/1
  In1/1 -> HwModeRegister1/1
  FS/1 -> PipelineRegister/1
  HwModeRegister/1 -> FS/1
  HwModeRegister1/1 -> FS/2

== system gm_RLUb_HIL/SignalMUX/AnalogOut/UnsignedScale ==
  In1 : Inport  OutDataTypeStr=fixdt(1, 25, 16)  PortDimensions=1  SampleTime=5e-08
  FS : Product  Inputs=**  OutDataTypeStr=fixdt(1, 50, 30)  SampleTime=5e-08
  FS_const : Constant  Value=524.28802490234375  OutDataTypeStr=fixdt(1, 25, 14)  SampleTime=-1
  FS_out_dtc : DataTypeConversion  OutDataTypeStr=uint16  SampleTime=5e-08  SaturateOnIntegerOverflow=on
  HwModeRegister : Delay  DelayLength=double(1)  InitialCondition=0  InputProcessing=Inherited  SampleTime=5e-08
  HwModeRegister1 : Delay  DelayLength=double(1)  InitialCondition=0  InputProcessing=Inherited  SampleTime=5e-08
  PipelineRegister : Delay  DelayLength=double(1)  InitialCondition=0  InputProcessing=Inherited  SampleTime=5e-08
  Out1 : Outport
  wires:
  FS_out_dtc/1 -> Out1/1
  FS_const/1 -> HwModeRegister/1
  PipelineRegister/1 -> FS_out_dtc/1
  In1/1 -> HwModeRegister1/1
  FS/1 -> PipelineRegister/1
  HwModeRegister/1 -> FS/1
  HwModeRegister1/1 -> FS/2

== system gm_RLUb_HIL/SignalMUX/AnalogOut/UnsignedScale1 ==
  In1 : Inport  OutDataTypeStr=fixdt(1, 25, 16)  PortDimensions=1  SampleTime=5e-08
  FS : Product  Inputs=**  OutDataTypeStr=fixdt(1, 50, 30)  SampleTime=5e-08
  FS_const : Constant  Value=524.28802490234375  OutDataTypeStr=fixdt(1, 25, 14)  SampleTime=-1
  FS_out_dtc : DataTypeConversion  OutDataTypeStr=uint16  SampleTime=5e-08  SaturateOnIntegerOverflow=on
  HwModeRegister : Delay  DelayLength=double(1)  InitialCondition=0  InputProcessing=Inherited  SampleTime=5e-08
  HwModeRegister1 : Delay  DelayLength=double(1)  InitialCondition=0  InputProcessing=Inherited  SampleTime=5e-08
  PipelineRegister : Delay  DelayLength=double(1)  InitialCondition=0  InputProcessing=Inherited  SampleTime=5e-08
  Out1 : Outport
  wires:
  FS_out_dtc/1 -> Out1/1
  FS_const/1 -> HwModeRegister/1
  PipelineRegister/1 -> FS_out_dtc/1
  In1/1 -> HwModeRegister1/1
  FS/1 -> PipelineRegister/1
  HwModeRegister/1 -> FS/1
  HwModeRegister1/1 -> FS/2
